simulink model "System_Tune"  (R2020b)
settings: Solver=VariableStepAuto  StartTime=0.0  StopTime=5  RelTol=1e-3
values from neighbouring files (symbols this model uses):
  Delay = 0.01e-4    (= 1e-06)    [PID_Tune.m]
  Den_Sys = [T 1]    [PID_Tune.m]
  Filter_Den = [L*C 0 1]    [PID_Tune.m]
  Filter_Num = [1]    [PID_Tune.m]
  Gain = 256/4096    (= 0.0625)    [PID_Tune.m]
  Num_Sys = [K]    [PID_Tune.m]
  PID_max = 4096    [PID_Tune.m]
  PID_min = 0    [PID_Tune.m]
  PWM_Period = 1e-3    (= 0.001)    [PID_Tune.m]
libraries: dsparch4 x2, simulink x2, pid_lib x1
settings Model: Creator=Arsalan_Ramzan_2  LastModifiedBy=Raheel J

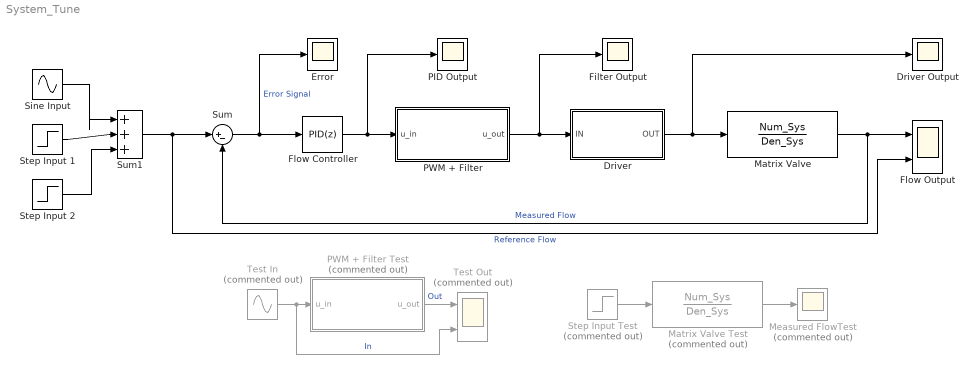
== system System_Tune ==
  Driver : Subsystem
  Driver Output : Scope
  Error : Scope
  Filter Output : Scope
  Flow Controller : pid_lib/PID Controller  Controller=PID  Form=Parallel  TimeDomain=Discrete-time  UseExternalTs=off  SampleTime=-1  IntegratorMethod=Forward Euler  FilterMethod=Forward Euler  ControllerParametersSource=internal  P=20  I=8000  D=0  UseFilter=on  N=100  TunerSelectOption=Transfer Function Based (PID Tuner App)  InitialConditionSource=internal  InitialConditionForIntegrator=0  InitialConditionForFilter=0  DifferentiatorICPrevScaledInput=0  ExternalReset=none  TrackingMode=off  Kt=1  LimitOutput=on  SatLimitsSource=internal  UpperSaturationLimit=PID_max  LowerSaturationLimit=PID_min  LinearizeAsGain=on  AntiWindupMode=none  Kb=1  POutMin=[]  POutMax=[]  IOutMin=[]  IOutMax=[]  DOutMin=[]  DOutMax=[]  NOutMin=[]  NOutMax=[]  SumOutMin=[]  SumOutMax=[]  SaturationOutMin=[]  SaturationOutMax=[]  PParamMin=[]  PParamMax=[]  IParamMin=[]  IParamMax=[]  DParamMin=[]  DParamMax=[]  NParamMin=[]  NParamMax=[]  KbParamMin=[]  KbParamMax=[]  KtParamMin=[]  KtParamMax=[]  KbOutMin=[]  KbOutMax=[]  KtOutMin=[]  KtOutMax=[]  IntegratorOutMin=[]  IntegratorOutMax=[]  FilterOutMin=[]  FilterOutMax=[]  SumI1OutMin=[]  SumI1OutMax=[]  SumI2OutMin=[]  SumI2OutMax=[]  SumI3OutMin=[]  SumI3OutMax=[]  SumI4OutMin=[]  SumI4OutMax=[]  SumDOutMin=[]  SumDOutMax=[]  DifferentiatorOutMin=[]  DifferentiatorOutMax=[]  FilterDiffOutCoefMin=[]  FilterDiffOutCoefMax=[]  ReciprocalOutMin=[]  ReciprocalOutMax=[]  SumDenOutMin=[]  SumDenOutMax=[]  SumNumOutMin=[]  SumNumOutMax=[]  DivideOutMin=[]  DivideOutMax=[]  UdiffTsProdOutMin=[]  UdiffTsProdOutMax=[]  NTsProdOutMin=[]  NTsProdOutMax=[]  UintegralTsProdOutMin=[]  UintegralTsProdOutMax=[]  UngainTsProdOutMin=[]  UngainTsProdOutMax=[]  IntegratorContinuousStateAttributes=''  IntegratorStateMustResolveToSignalObject=off  IntegratorRTWStateStorageClass=Auto  FilterContinuousStateAttributes=''  FilterStateMustResolveToSignalObject=off  FilterRTWStateStorageClass=Auto  ParallelPVariant=InternalParameters  IdealPVariant=Disabled  IVariant=InternalParameters  DVariant=InternalParameters  IntegratorVariant=Discrete  SatVariant=Enabled  AWVariant=Passthrough  PCopyVariant=Disabled  TRVariant=Disabled  FdbkBlocksVariant=Forward  IdealPFdbkVariant=Disabled  SatFdbkVariant=Disabled  DerivativeFilterVariant=ForwardEulerFilter  NVariant=InternalParameters  NCopyVariant=Disabled  FilterICVariant=InternalICsFilter  IntegratorICVariant=InternalICs  ExternalResetVariant=Disabled  TRSumVariant=Passthrough  SumFdbkVariant=Disabled  SumVariant=Sum_PID  TsampFilterVariant=InternalTs  TsampNgainVariant=Passthrough  TsampIntegralVariant=Passthrough  ExternalSaturationOutDataTypeStr=Inherit: Same as second input
  Flow Output : Scope  NumInputPorts=2
  Matrix Valve : TransferFcn  Numerator=Num_Sys  Denominator=Den_Sys
  Matrix Valve Test : TransferFcn  Commented=on  Numerator=Num_Sys  Denominator=Den_Sys
  Measured FlowTest : Scope  Commented=on
  PID Output : Scope
  PWM + Filter : Subsystem
  PWM + Filter Test : Subsystem  Commented=on
  Sine Input : Sin  Amplitude=5  Bias=5  Frequency=10  SampleTime=0
  Step Input 1 : Step  Time=0.5  After=50  SampleTime=0
  Step Input 2 : Step  Time=3  After=-30  SampleTime=0
  Step Input Test : Step  Commented=on  After=50  SampleTime=0
  Sum : Sum  Inputs=|+-
  Sum1 : Sum  Inputs=|+++
  Test In : Sin  Commented=on  Amplitude=0.5  Bias=0.5  Frequency=24  SampleTime=0
  Test Out : Scope  Commented=on  NumInputPorts=2
  wires:
  Flow Controller/1 -> PWM + Filter/1(u_in), PID Output/1
  Sum/1 -> Error/1, Flow Controller/1  "Error Signal"
  Matrix Valve/1 -> Flow Output/1, Sum/2  "Measured Flow"
  PWM + Filter/1(u_out) -> Driver/1(IN), Filter Output/1
  Sum1/1 -> Flow Output/2, Sum/1  "Reference Flow"
  Test In/1 -> Test Out/2, PWM + Filter Test/1(u_in)  "In"
  PWM + Filter Test/1(u_out) -> Test Out/1  "Out"
  Driver/1(OUT) -> Matrix Valve/1, Driver Output/1
  Matrix Valve Test/1 -> Measured FlowTest/1
  Step Input Test/1 -> Matrix Valve Test/1
  Step Input 2/1 -> Sum1/3
  Step Input 1/1 -> Sum1/2
  Sine Input/1 -> Sum1/1

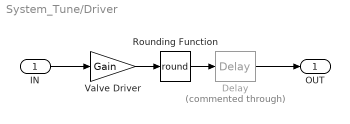
== system System_Tune/Driver ==
  IN : Inport
  Delay : TransportDelay  Commented=through  DelayTime=Delay  BufferSize=1024e2
  Rounding Function : Rounding  Operator=round
  Valve Driver : Gain  Gain=Gain
  OUT : Outport
  wires:
  Rounding Function/1 -> Delay/1
  Valve Driver/1 -> Rounding Function/1
  Delay/1 -> OUT/1
  IN/1 -> Valve Driver/1

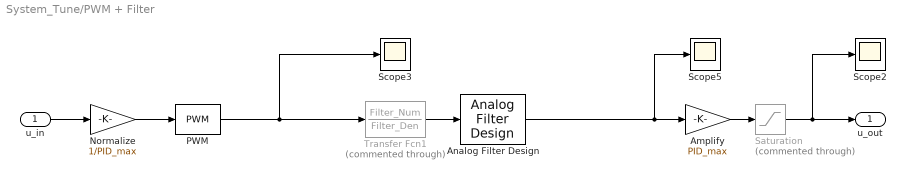
== system System_Tune/PWM + Filter ==
  u_in : Inport
  Amplify : Gain  Gain=PID_max
  Analog Filter Design : dsparch4/Analog Filter Design  method=Butterworth  filttype=Lowpass  N=2  Wlo=1000  Whi=80  Rp=2  Rs=40
  Normalize : Gain  Gain=1/PID_max
  PWM : simulink/Discontinuities/PWM  DisableCoverage=on  Period=PWM_Period  DisallowZeroDutyCycle=off  RunAtFixedTimeIntervals=on  SampleTime=1e-6
  Saturation : Saturate  Commented=through  UpperLimit=PID_max  LowerLimit=PID_min
  Scope2 : Scope
  Scope3 : Scope
  Scope5 : Scope
  Transfer Fcn1 : TransferFcn  Commented=through  Numerator=Filter_Num  Denominator=Filter_Den
  u_out : Outport
  wires:
  Transfer Fcn1/1 -> Analog Filter Design/1
  Saturation/1 -> u_out/1, Scope2/1
  PWM/1 -> Scope3/1, Transfer Fcn1/1
  u_in/1 -> Normalize/1
  Normalize/1 -> PWM/1
  Amplify/1 -> Saturation/1
  Analog Filter Design/1 -> Scope5/1, Amplify/1

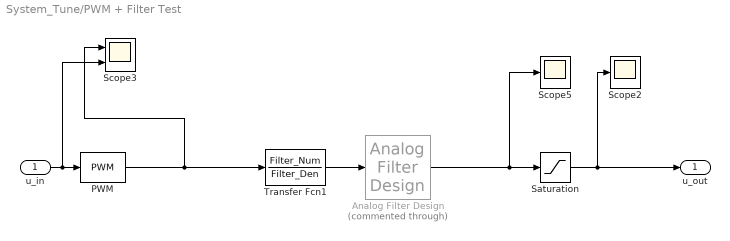
== system System_Tune/PWM + Filter Test ==
  u_in : Inport
  Analog Filter Design : dsparch4/Analog Filter Design  Commented=through  method=Butterworth  filttype=Lowpass  N=2  Wlo=3000  Whi=80  Rp=2  Rs=40
  PWM : simulink/Discontinuities/PWM  DisableCoverage=on  Period=PWM_Period  DisallowZeroDutyCycle=off  RunAtFixedTimeIntervals=off  SampleTime=1e-6
  Saturation : Saturate  UpperLimit=PID_max  LowerLimit=PID_min
  Scope2 : Scope
  Scope3 : Scope  NumInputPorts=2
  Scope5 : Scope
  Transfer Fcn1 : TransferFcn  Numerator=Filter_Num  Denominator=Filter_Den
  u_out : Outport
  wires:
  u_in/1 -> Scope3/2, PWM/1
  PWM/1 -> Transfer Fcn1/1, Scope3/1
  Saturation/1 -> Scope2/1, u_out/1
  Transfer Fcn1/1 -> Analog Filter Design/1
  Analog Filter Design/1 -> Saturation/1, Scope5/1
